simulink model "DMS_Master"  (Simulink 8.1)
settings: Solver=ode3  StartTime=0.0  StopTime=10.0  FixedStep=Ts  RelTol=1e-3
PostLoadFcn:
  | Ts=100e-6; HILLTOP_init;SIM_HIL=0; UnitTest_Breaker_init
InitFcn:
  | Ts=100e-6; HILLTOP_init;SIM_HIL=0; UnitTest_Breaker_init
values from neighbouring files (symbols this model uses):
  CMD_signals = [0 300 600 900 1200 1500 1800 2100 2400 2700 3000 3300 ... (1568 elements, 49x32)]    [CMD_signals.mat]
libraries: artemis x1, powerlib x1
settings Model: ARTEMISmethode_block_infos=$$__separator__$$DMS_Master/ARTEMIS Guide$$__separator__$$  Creator=ed12083  LastModifiedBy=ed12083
settings DataIOCC: SignalLoggingSaveFormat=Dataset
settings OptimizationCC: ExpressionDepthLimit=128
settings DebuggingCC: FcnCallInpInsideContextMsg=EnableAllAsError
settings GRTTargetCC: CombineOutputUpdateFcns=on  GRTInterface=off

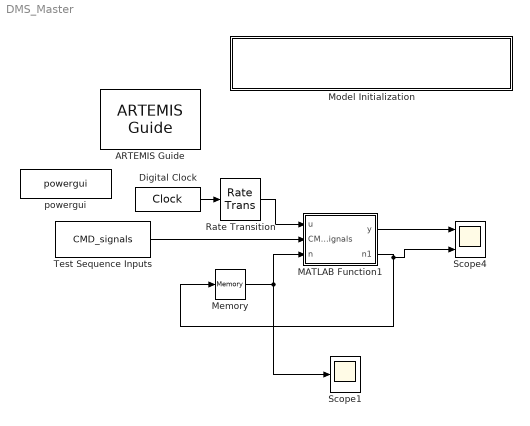
== system DMS_Master ==
  ARTEMIS Guide : artemis/ARTEMIS/ARTEMIS Guide  Tag=FTSSmethode_opal_4hx0r99  Description=5.0_z1  lock=on  Ts=Ts  opt=art5  dyna=off  nb_perm=4  RT_fullcomp=off  ssn=on  ssn_itvc=off  ssn_ivic=off  ssn_ext=off  ssn_solver=Art5 with Backward Euler nodal interface  ssn_impulse=off  ssn_quasimpulse=off  ssn_impulse_loop=2  paraExtinctionThy=off  Thy_Impulse=on  dtc=Off  dtc_opt=normal  ao=on  simtype=off  ct_mac=off  lin_mov=off  lsp=[0.001 2]  spike_skip=Disabled  dtc_extra=1  dtc_sws=normal  dtc_pied=0.5  SPSRulesBlock=SPSRules  tre=on  ctmm=off  LF=off  dpl_type=ARTEMiS DPL  rlc_type=off  custom_type=off  para=on  ssn_ImpulseLoopBlockedStateUpdate=2  ssn_mov_iter_number=5  ssn_switch_iter_number=5
  Digital Clock : DigitalClock
  MATLAB Function1 : MATLAB Function  TreatAsAtomicUnit=on
  Memory : Memory  X0=1
  Model Initialization : Subsystem  AncestorBlock=artemis/Tools /Misc/Model Initialization  mask(Model Functions){InitFcnX=Ts=100e-6; HILLTOP_init;SIM_HIL=0; UnitTest_Breaker_init, prel=off, posl=on, inif=on, strf=off}
      mask prompts: InitFcnX "Initialisation"; prel "Preload Function"; posl "PostLoad Function"; inif "InitFcn"; strf "StartFcn"
      mask init:
      | currentBlock = gcb;
      | root = bdroot(currentBlock);
      | 
      | 
      | if ~strcmp(get_param(root,'BlockDiagramType'),'library')
      |     if prel==1
      |         set_param(root, 'PreLoadFcn', InitFcnX);
      |     else
      |         set_param(root, 'PreLoadFcn', '');
      |     end
      |     if inif==1
      |         set_param(root, 'InitFcn', InitFcnX);
      |     else
      |         set_param(root, 'InitFcn', '');
      |     end
      |     if strf==1
      |         set_param(root, 'StartFcn', InitFcnX);
      |     else
      |         set_param(root, 'StartFcn', '');
      |     end
      |     if posl==1
      |         set_param(root, 'PostLoadFcn', InitFcnX);
      |     else
      |         set_param(root, 'PostLoadFcn', '');
      |     end
      | end
      | 
      | pos = get_param(currentBlock, 'Position');
      | width = pos(3) - pos(1); height = pos(4) - pos(2);
      | txt = [ upper(root) '\n' '- InitFcn. . . . . '  get_param(root, 'InitFcn') ];
      settings: CopyFcn=set_param(gcb,'LinkStatus','inactive')
      mask Display: text(5, height*0.5, txt, 'horizontalAlignment', 'left', 'verticalAlignment', 'middle') ;
  Rate Transition : RateTransition
  Scope1 : Scope
  Scope4 : Scope  NumInputPorts=3
      settings: YMin=-5~-5~-5  YMax=5~5~5
  Test Sequence Inputs : Constant  Value=CMD_signals
  powergui : powerlib/powergui  Priority=2  SimulationMode=Discrete  SolverType=Tustin  SampleTime=Ts  frequency=60  SPID=off  DisableSnubberDevices=off  DisableRonSwitches=off  DisableVfSwitches=off  SwTol=0  Interpol=off  DisplayEquations=off  frequencyindice=0  Pbase=100e6  ErrMax=1e-4  Iterations=50  UnitsV=kV  UnitsW=MW  FunctionMessages=off  echomessages=off  HookPort=off  EnableUseOfTLC=off  x0status=blocks  RestoreLinks=warning  ResistiveCurrentMeasurement=off  Frange=logspace(0,3,50)  Ylog=off  Xlog=off  ShowGrid=off  save=off  variable=ZData  structure=0  ZoomFFT=on  StartTime=0.0  cycles=2  DisplayStyle=off  fundamental=60  FreqAxis=off  MaxFrequency=1000  frequencyindicesteady=1  RmsSteady=1  display=off  Ts=0  methode=off
  wires:
  Digital Clock/1 -> Rate Transition/1
  MATLAB Function1/1(y) -> Scope4/1
  MATLAB Function1/2(n1) -> Memory/1, Scope4/3
  Memory/1 -> MATLAB Function1/3(n), Scope1/1
  Test Sequence Inputs/1 -> MATLAB Function1/2(CMD_signals)
  Rate Transition/1 -> MATLAB Function1/1(u)

== system DMS_Master/Model Initialization ==

== matlab function MATLAB Function1 ==
  data: u input double; y output double; CMD_signals input double; n input double; n1 output double
function [y,n1] = fcn(u,CMD_signals,n)
% Author: Matthew Backes, MIT Lincoln Laboratory
% Date: 8/16/2016
%
% Edited 9/6/2016 by E. Corbett to remove repeated Modbus register 0007 for
% DSO Import value
%
% This function takes in the test sequence signals from a .mat file which
% is generated with the ____.m script. It then updates the parameters
% within the simulink model according to the time stamp of the test
% sequence command signals.
% CMD column 1 = time
% CMD column 2 = POI feeder 1 SEL relay
% CMD column 3 = POI feeder 2 SEL relay
% CMD column 4 = POI feeder 3 SEL relay
% CMD column 5 = diesel breaker
% CMD column 6 = solar irradiance gain
% CMD column 7 = solar breaker
% CMD column 8 = CHP breaker
% CMD column 9 = load gain
% CMD column 10 = motor 1 breaker
% CMD column 11 = motor 2 breaker
% CMD column 12 = fault location 1
% CMD column 13 = fault location 2
% CMD column 14 = fault location 3
% CMD column 15 = fault location 4
% CMD column 16 = fault location 5
% CMD column 17 = fault location 6
% CMD column 18 = fault location 7
% CMD column 19 = fault location 8 SECT
%
%NEXT
% CMD column 20 = dso Disconnect command
% CMD column 21 = dso Reconnect command
% CMD column 22 = dso Export command
% CMD column 23 = dso Import command
% CMD column 24 = dso power factor command
% CMD column 25 = dso VAR support command
% CMD column 26 = dso Demand Response command
% CMD column 27 = dso Import/export value
% CMD column 28 = dso power factor value
% CMD column 29 = dso VAR value
% CMD column 30 = dso DR value
% CMD column 31 = dso Command start time
% CMD column 32 = dso command duration

y = u;

coder.extrinsic('set_param') %declare set_param as an extrinsic function
coder.extrinsic('num2str') %declare num2str as an extrinsic function
coder.extrinsic('tcpip')

time = CMD_signals(:,1); 
%time_lastCMD = time(length(time)); %do i need this anymore?
numCMDs = length(time);
DMS_ipaddr = '192.168.10.40';
%DMS_ipaddr = '127.0.0.1';
POI_F1_ipaddr = '192.168.10.41';
POI_F2_ipaddr = '192.168.10.42';
POI_F3_ipaddr = '192.168.10.43';
port = 512;

handles=tcpip(DMS_ipaddr, port,'Timeout',1);    %Create the tcpip object
set(handles, 'InputBufferSize', 512);       %assign the buffer
set(handles, 'ByteOrder', 'bigEndian');              %specify the order in which bytes are transmitted

% set(handles, 'Connected', 0);                            %default is not connected
% try 
Status=get(handles, 'Status');
%    if ~strcmp(Status,'open')       %if not open then 
%        Tcp=get(handles, 'tcp');
        fopen(handles);                     %open a connection
%        set(handles, 'connected', 1);                   %connected
%    end


if n > numCMDs   %do nothing if we have exhausted all commands
    n1 = n;
else
    if u > time(n) % when the simulation time is greater than the command signal time, execute set_param
        n1 = n+1; % increment to next command to execute
        
        %parameters to set within simulink model
        set_param('testScript_model/TestCommands','diesel_breaker',num2str(CMD_signals(n,5)),'pv_breaker',num2str(CMD_signals(n,7)),'CHP_breaker',num2str(CMD_signals(n,8)),'load_gain',num2str(CMD_signals(n,9)),'motor1_breaker',num2str(CMD_signals(n,10)),'motor2_breaker',num2str(CMD_signals(n,11)),'fault1',num2str(CMD_signals(n,12)),'fault2',num2str(CMD_signals(n,13)),'fault3',num2str(CMD_signals(n,14)),'fault4',num2str(CMD_signals(n,15)),'fault5',num2str(CMD_signals(n,16)),'fault6',num2str(CMD_signals(n,17)),'fault7',num2str(CMD_signals(n,18)),'fault8',num2str(CMD_signals(n,19)));
        
        %modbus commands
%         if CMD_signals(n,2) == 1    %if 1, then POI_1 should be open -> issue Modbus command
%             ctrl_device_DMS_modbus(POI_F1_ipaddr,502,[20,0,6,1,6,hex2dec('2000'),2]);
%         else
%             ctrl_device_DMS_modbus(POI_F1_ipaddr,502,[20,0,6,1,6,hex2dec('2001'),1]);
%         end
%         if CMD_signals(n,3) == 1
%             ctrl_device_DMS_modbus(POI_F2_ipaddr,502,[20,0, 6, 1, 6, 2000, 2]);
%         else
%             ctrl_device_DMS_modbus(POI_F2_ipaddr,502,[20,0,6,1,6,2001,1]);
%         end
%         if CMD_signals(n,4) == 1
%             ctrl_device_DMS_modbus(POI_F3_ipaddr,502,[20,0,6,1,6,2000,2]);
%         else
%             ctrl_device_DMS_modbus(POI_F3_ipaddr,502,[20,0,6,1,6,2001,1]);
%         end
%         
%         if dsoDisconnect(n) == 1 
%             ctrl_device_DMS_modbus(DMS_ipaddr,502,[10, 0, 6, 1, 6, 0000, 1]); %do i need to reset this?
%         end
%         if dsoReconnect(n) == 1 
%             ctrl_device_DMS_modbus(DMS_ipaddr,502,[10, 0, 6, 1, 6, 0001, 1]);
%         end
%         if dsoExport(n) == 1
%             ctrl_device_DMS_modbus(DMS_ipaddr,502,[10, 0, 6, 1, 6, 0002, 1]);
%             ctrl_device_DMS_modbus(DMS_ipaddr,502,[10, 0, 6, 1, 6, 0007, CMD_Signals(n,27)]);
%         end
%         if dsoImport(n) == 1
%             ctrl_device_DMS_modbus(DMS_ipaddr,502,[10, 0, 6, 1, 6, 0003, 1]);
%             ctrl_device_DMS_modbus(DMS_ipaddr,502,[10, 0, 6, 1, 6, 0008, CMD_Signals(n,27)]);
%         end
%         if dsoPF(n) == 1 
%             ctrl_device_DMS_modbus(DMS_ipaddr,502,[10, 0, 6, 1, 6, 0004, 1]);
%             ctrl_device_DMS_modbus(DMS_ipaddr,502,[10, 0, 6, 1, 6, 0009, CMD_Signals(n,28)]);
%         end
%         if dsoVAR(n) == 1
%             ctrl_device_DMS_modbus(DMS_ipaddr,502,[10, 0, 6, 1, 6, 0005, 1]);
%             ctrl_device_DMS_modbus(DMS_ipaddr,502,[10, 0, 6, 1, 6, 0010, CMD_Signals(n,29)]);
%         end
%         if dsoDR(n) == 1
%             ctrl_device_DMS_modbus(DMS_ipaddr,502,[10, 0, 6, 1, 6, 0006, 1]);
%             ctrl_device_DMS_modbus(DMS_ipaddr,502,[10, 0, 6, 1, 6, 0011, CMD_Signals(n,30)]);
%         end
%         
%         ctrl_device_DMS_modbus(DMS_ipaddr,502,[10, 0, 6, 1, 6, 0012, u]);
%         ctrl_device_DMS_modbus(DMS_ipaddr,502,[10, 0, 6, 1, 6, 0013, CMD_Signals(n,31)]);
%         ctrl_device_DMS_modbus(DMS_ipaddr,502,[10, 0, 6, 1, 6, 0014, CMD_Signals(n,32)]);
        
     else  % wait until the simulation time has eclisped the next command time
        n1 = n; 
    end
end
